simulink library "orion_casestudy_1_1"  (R2023a)
settings: Solver=ode45  StartTime=0.0  StopTime=10.0  RelTol=1e-3  AbsTol=1e-6
settings Model: ExtModeTrigMode=oneshot  Creator=The MathWorks, Inc.  LastModifiedBy=simon
settings SolverCC: AutoScaleAbsTol=off  AlgebraicLoopSolver=TrustRegion
settings DataIOCC: SaveFormat=Array  SignalLoggingSaveFormat=ModelDataLogs  ReturnWorkspaceOutputs=off  SignalLoggingName=logsOut
settings OptimizationCC: BooleanDataType=off  ReuseModelBlockBuffer=off  ExpressionDepthLimit=2147483647  InitFltsAndDblsToZero=on  EfficientMapNaN2IntZero=off  LifeSpan=inf  BufferReusableBoundary=off
settings DebuggingCC: SaveWithParameterizedLinksMsg=none  UnderspecifiedInitializationDetection=Classic  MergeDetectMultiDrivingBlocksExec=none  CheckExecutionContextPreStartOutputMsg=on  SignalResolutionControl=TryResolveAllWithWarning  MultiTaskDSMMsg=warning  MultiTaskCondExecSysMsg=none  IntegerOverflowMsg=none  FcnCallInpInsideContextMsg=warning  UnconnectedInputMsg=warning  UnconnectedOutputMsg=warning  UnconnectedLineMsg=warning  AllowSymbolicDim=off  StateNameClashWarn=warning  SFUnexpectedBacktrackingDiag=warning  SFNoUnconditionalDefaultTransitionDiag=warning  SFExecutionAtInitializationDiag=none  IntegerSaturationMsg=none  ArithmeticOperatorsInVariantConditions=warning
settings HardwareCC: ProdBitPerPointer=32  ProdLargestAtomicFloat=None  ProdIntDivRoundTo=Undefined  ProdEndianess=Unspecified  ProdWordSize=32  ProdHWDeviceType=32-bit Generic  TargetUnknown=on
settings ModelReferenceCC: UpdateModelReferenceTargets=IfOutOfDate  EnableRefExpFcnMdlSchedulingChecks=on  PropagateSignalLabelsOutOfModel=off
settings SFSimCC: SimUseLocalCustomCode=off  CustomCodeUndefinedFunction=UseInterfaceOnly
settings RTWCC: RTWUseLocalCustomCode=off  DLArmComputeVersion=19.05
settings CodeAppCC: StateflowObjectComments=on
settings GRTTargetCC: TargetFcnLib=ansi_tfl_tmw.mat  TargetLangStandard=C89/C90 (ANSI)  CombineOutputUpdateFcns=off  GRTInterface=on
settings ConfigComp: CovMetricSettings=dw  CovSaveCumulativeToWorkspaceVar=on  CovSaveSingleToWorkspaceVar=on  CovExternalEMLEnable=off  CovSFcnEnable=off

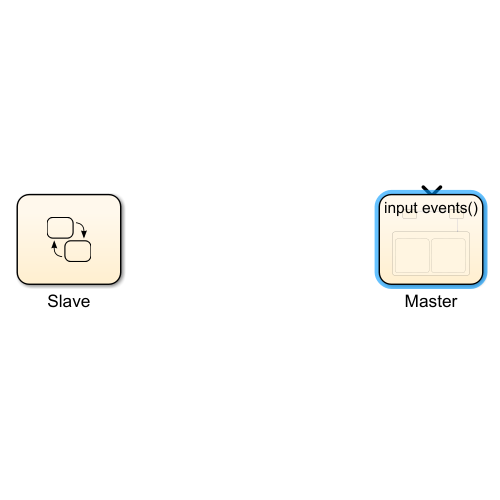
[thumbnail: Simulink's stored preview of the top-level diagram]
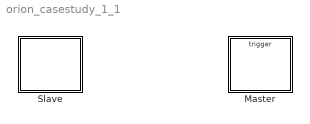
== system orion_casestudy_1_1 ==
  Master : Stateflow chart  BlockKeywords=__PRM__SERIALIZED__DATA__:Stateflow Chart,Stateflow Diagram  TreatAsAtomicUnit=on
  Slave : Stateflow chart  TreatAsAtomicUnit=on

== stateflow chart orion_casestudy_1_1/Slave ==

== stateflow chart orion_casestudy_1_1/Master ==
  note: OrionDisconn
  state Closed_0
  state Connecting_2
  state Connected_4
    state KeepAliveSendTimeout_1 [parallel]
      settings: executionOrder=2
    state region_2_in_Kapcsolodva_4 [parallel]
      settings: executionOrder=1
  (default) -> Closed_0
  Closed_0 -> Connecting_2
  Connecting_2 -> Connected_4
  events: OrionDisconnIn input FUNCTION_CALL_EVENT; OrionAppDataIn input FUNCTION_CALL_EVENT; OrionConnReqIn input FUNCTION_CALL_EVENT; OrionDisconnCauseIn input FUNCTION_CALL_EVENT; OrionConnConfIn input FUNCTION_CALL_EVENT; OrionConnRespIn input FUNCTION_CALL_EVENT; OrionKeepAliveIn input FUNCTION_CALL_EVENT; OrionDisconnOut input FUNCTION_CALL_EVENT; OrionDisconnCauseOut input FUNCTION_CALL_EVENT; OrionConnReqOut input FUNCTION_CALL_EVENT; OrionAppDataOut input FUNCTION_CALL_EVENT; OrionKeepAliveOut input FUNCTION_CALL_EVENT; OrionConnConfOut input FUNCTION_CALL_EVENT; OrionConnRespOut input FUNCTION_CALL_EVENT
